simulink model "Final_Model_Building_2_AirflowAdded"  (R2022a)
settings: Solver=ode1  StartTime=0.0  StopTime=24*3600  FixedStep=10  RelTol=1e-3
values from neighbouring files (symbols this model uses):
  Aux_Threshold = 52    [Setup_Code_EWASP_VC.m]
  buildingAge = 2005    [Setup_Code_EWASP_VC.m]
  ceilingHeight = 2.4    [Setup_Code_EWASP_VC.m]
  conductiveHconnectMatrix = [ ... (first row only)    [Setup_Code_EWASP_VC.m]
  cRoofGreen = 100000    [Setup_Code_EWASP_VC.m]
  Defrost_After_Time = 30    [Setup_Code_EWASP_VC.m]
  DHWDemandProfile = occFreegainHotwaterElecTestPassiveOcc3(:,3)    [Setup_Code_EWASP_VC.m]
  Elec_Max = Elec_Max*(30/24.2)    [Setup_Code_EWASP_VC.m]
  Elec_Mid = Elec_Mid*(30/24.2)    [Setup_Code_EWASP_VC.m]
  Elec_Min = Elec_Min*(30/24.2)    [Setup_Code_EWASP_VC.m]
  ElecDemandProfile = occFreegainHotwaterElecTestPassiveOcc3(:,4)    [Setup_Code_EWASP_VC.m]
  ElecFixed = [Elec_Max(6,2) Elec_Max(6,4) Elec_Max(6,6) Elec_Max(6,7) ... (first row only)    [Setup_Code_EWASP_VC.m]
  floorOrCeilingArea = floorOrCeilingArea*1.15    [Setup_Code_EWASP_VC.m]
  forceCold = 0    [Setup_Code_EWASP_VC.m]
  freegain = occFreegainHotwaterElecTestPassiveOcc3(:,2)-max(occupancy)*25    [Setup_Code_EWASP_VC.m]
  furnitureModelOn = 1    [Setup_Code_EWASP_VC.m]
  Heat_Max = Heat_Max*(30/24.2)    [Setup_Code_EWASP_VC.m]
  Heat_Mid = Heat_Mid*(30/24.2)    [Setup_Code_EWASP_VC.m]
  Heat_Min = Heat_Min*(30/24.2)    [Setup_Code_EWASP_VC.m]
  HeatFixed = [Heat_Max(6,2) Heat_Max(6,4) Heat_Max(6,6) Heat_Max(6,7) ... (first row only)    [Setup_Code_EWASP_VC.m]
  HeatingOnProfile = repmat(HeatingOnProfile,365,1)    [Setup_Code_EWASP_VC.m]
  HEX_ReturnLowerLimit = 52.5    [Setup_Code_EWASP_VC.m]
  HEX_ReturnUpperLimit = 55    [Setup_Code_EWASP_VC.m]
  LeakMultiplier = 1+(2*(rand()-0.5)/10)    [Setup_Code_EWASP_VC.m]
  maxOcc = max(occupancyProfile)    [Setup_Code_EWASP_VC.m]
  NESW_wallArea = max(NESW_Lengths*ceilingHeight-NESW_Windows,0)    [Setup_Code_EWASP_VC.m]
  NESW_Windows = [ ... (first row only)    [Setup_Code_EWASP_VC.m]
  numRooms = roomCount    [Setup_Code_EWASP_VC.m]
  occupancy = occupancyProfile    [Setup_Code_EWASP_VC.m]
  offsetDays = 0    [Setup_Code_EWASP_VC.m]
  pumpChoice = pumpChoices(MinIndex,1)    [Setup_Code_EWASP_VC.m]
  pumpRamp = 180    [Setup_Code_EWASP_VC.m]
  ReturnLowerLimit = 37.5    [Setup_Code_EWASP_VC.m]
  ReturnUpperLimit = 40    [Setup_Code_EWASP_VC.m]
  RoofIrradiance = Flat_NS_EW_RoofIrradiance(:,1)    [Setup_Code_EWASP_VC.m]
  roofStartTemp = ones(11,1)*20    [Setup_Code_EWASP_VC.m]
  rooftype = 0    [Setup_Code_EWASP_VC.m]
  RoomDataMatrix = [zeros(1,12);ones(1,12)*wallDensity;zeros(1,12);ones(1,12)*wallU;ones(1,12)*windowU;ones(1,12)*floorU;ones(1,12)*ceilingU;zeros(1,12);windowArea, 0;floorOrCeilingArea;zeros(1,12);floorOrCeilingArea*ceilingHeight]    [Setup_Code_EWASP_VC.m]
  roomVol = roomVol*1.15    [Setup_Code_EWASP_VC.m]
  slabStartTemp = (GroundTempTimeSeries(offsetDays*1440+1,1)+thermostatSetting)/2    [Setup_Code_EWASP_VC.m]
  SlackRequest = zeros(1440,1)    [Setup_Code_EWASP_VC.m]
  SolarThermalExists = 0    [Setup_Code_EWASP_VC.m]
  SourceFixed = HeatFixed-ElecFixed    [Setup_Code_EWASP_VC.m]
  StateSeries = StateSeriesGenerator(22,7,1)    [Setup_Code_EWASP_VC.m]
  Tank_Lower_Temp = 49.5    [Setup_Code_EWASP_VC.m]
  Tank_Upper_Temp = 52    [Setup_Code_EWASP_VC.m]
  Tank_Volume_m3 = 0.15    [Setup_Code_EWASP_VC.m]
  TankHeatHour = randi([1 5])-1    [Setup_Code_EWASP_VC.m]
  upDown = [0;0;0;0;1;1;1;1;1;1;1]    [Setup_Code_EWASP_VC.m]
  wallStartTempExt = thermostatSetting*(0.266+0.00215*outdoorStartTemp+0.018*wallU+0.00113*outdoorStartTemp*wallU+0.0068*wallU^2)    [Setup_Code_EWASP_VC.m]
undefined symbols (not defined in the file or in its folder): a, ceilingU, condUDMatrix, convUDMatrix, deltaPEXPANDED_E, deltaPEXPANDED_E2, deltaPEXPANDED_N, deltaPEXPANDED_N2, deltaPEXPANDED_S, deltaPEXPANDED_S2, deltaPEXPANDED_W, deltaPEXPANDED_W2, DesiredDHWTemp, DesiredFlowTempVsInOutDeltaTemp, DiffuseHorizontal, DiscIntNeverNeededParam, DNI, dwnAndConcrete, DWORK_A_HX, DWORK_CHK_FLU, DWORK_CP_NODE, DWORK_DH, DWORK_FLUID, DWORK_HCON, DWORK_LOSS, DWORK_MDOTDOWN, DWORK_MDOTIN, DWORK_MDOTUP, DWORK_MIX, DWORK_PRESS, DWORK_QDOTIN, DWORK_RHO_NODE, DWORK_TIN, DWORK_TS_OLD, DWORK_V_NODE, ExtractRates, GroundTempTimeSeries, HCM, HCM2, HCM_closed, HCM_closed2, intermediateU, IsTop, massFlowMatrix, mechEfficiency, neighbourMatrix, numericalRoomUse, RadiatorMatrix, room2roomflowmatrix_E, room2roomflowmatrix_E2, room2roomflowmatrix_N, room2roomflowmatrix_N2, room2roomflowmatrix_S, room2roomflowmatrix_S2, room2roomflowmatrix_W, room2roomflowmatrix_W2, StateAirInEXPANDED_E, StateAirInEXPANDED_E2, StateAirInEXPANDED_N, StateAirInEXPANDED_N2 ... (+27)
libraries: simulink x6, dspsigops x4, dspmtrx3 x4, carnot x3, spsEdgeDetectorLib x2, dspstat3 x2, powerlib_meascontrol x1, simulink_extras x1
(part 2 of 27)

== system Final_Model_Building_2_AirflowAdded/Airflow Model ==
  note: Select the correct state solution from
      | the 2 states that are simulated
  In1 : Inport
  In2 : Inport  Port=2
  In3 : Inport  Port=3
  In4 : Inport  Port=4
  In5 : Inport  Port=5
  " output 1 - air is coming in output 2 - air is going out" : Subsystem
  Constant : Constant  Value=ExtractRates
  Constant1 : Constant  Value=occupancy
  Constant10 : Constant  Value=StateAirInEXPANDED_S
  Constant11 : Constant  Value=StateAirInEXPANDED_W
  Constant12 : Constant  Value=StateAirOutEXPANDED_S
  Constant13 : Constant  Value=StateAirOutEXPANDED_W
  Constant14 : Constant  Value=StateAirOutEXPANDED_N
  Constant15 : Constant  Value=StateAirOutEXPANDED_E
  Constant16 : Constant  Value=deltaPEXPANDED_N
  Constant17 : Constant  Value=deltaPEXPANDED_E
  Constant18 : Constant  Value=deltaPEXPANDED_S
  Constant19 : Constant  Value=deltaPEXPANDED_W
  Constant2 : Constant  Value=roomVol
  Constant20 : Constant  Value=numRooms
  Constant21 : Constant  Value=buildingAge
  Constant22 : Constant  Value=0
  Constant23 : Constant  Value=StateAirInEXPANDED_S2
  Constant24 : Constant  Value=StateAirInEXPANDED_W2
  Constant25 : Constant  Value=StateAirOutEXPANDED_S2
  Constant26 : Constant  Value=StateAirOutEXPANDED_W2
  Constant27 : Constant  Value=StateAirOutEXPANDED_N2
  Constant28 : Constant  Value=StateAirOutEXPANDED_E2
  Constant29 : Constant  Value=deltaPEXPANDED_N2
  Constant3 : Constant  Value=buildingAge
  Constant30 : Constant  Value=deltaPEXPANDED_E2
  Constant31 : Constant  Value=deltaPEXPANDED_S2
  Constant32 : Constant  Value=deltaPEXPANDED_W2
  Constant33 : Constant  Value=[0;0;0;0;0;0;0;0;0;0;0]
  Constant34 : Constant  Value=numRooms
  Constant35 : Constant  Value=[0;0;0;0;0;0;0;0;0;0;0]
  Constant36 : Constant  Value=room2roomflowmatrix_N2
  Constant37 : Constant  Value=room2roomflowmatrix_E2
  Constant38 : Constant  Value=room2roomflowmatrix_S2
  Constant39 : Constant  Value=room2roomflowmatrix_W2
  Constant4 : Constant  Value=room2roomflowmatrix_N
  Constant40 : Constant  Value=StateAirInEXPANDED_N2
  Constant41 : Constant  Value=StateAirInEXPANDED_E2
  Constant42 : Constant  Value=[0;0;0;0;0;0;0;0;0;0;0]
  Constant5 : Constant  Value=room2roomflowmatrix_E
  Constant6 : Constant  Value=room2roomflowmatrix_S
  Constant7 : Constant  Value=room2roomflowmatrix_W
  Constant8 : Constant  Value=StateAirInEXPANDED_N
  Constant9 : Constant  Value=StateAirInEXPANDED_E
  Corrected buoyancy2 : Display  Commented=on
  Corrected buoyancy3 : Display  Commented=on
  IsNaN : RelationalOperator  Operator=isNaN  OutDataTypeStr=boolean  RndMeth=Simplest  InputSameDT=off
  MATLAB Function : MATLAB Function  TreatAsAtomicUnit=on
  MATLAB Function1 : MATLAB Function  TreatAsAtomicUnit=on
  MATLAB Function2 : MATLAB Function  TreatAsAtomicUnit=on
  Mean : dspstat3/Mean  run=off  InputProcessing=Columns as channels (frame based)  reset_popup=None  directionMode=Each column  dimension=1  roiEnable=off  roiType=Rectangles  roiPortion=Entire ROI  roiOutput=Individual statistics for each ROI  roiFlag=off  roundingMode=Floor  overflowMode=off  outputDataTypeStr=Inherit: Same as accumulator  outputMin=[]  outputMax=[]  outputLastDataTypeStr=Inherit: Same as accumulator
  Offset Independent time series element selector2 : Subsystem
  Permute Dimensions : PermuteDimensions
  Plus{,2..3,5} (4 alike) : Sum
  Plus1 : Sum  Inputs=+-
  Plus4 : Sum  Inputs=+-
  Product1 : Product
  Product10 : Product  Inputs=*/
  Product2 : Product  Inputs=4
  Product3 : Product  Inputs=4
  Product4 : Product  Inputs=*/
  Product5 : Product  Inputs=**
  Product6 : Product  Inputs=**
  Product9 : Product
  Rate Transition{,1..5} (6 alike) : RateTransition  OutPortSampleTime=900
  Relay1 : Relay  OnSwitchValue=ThermostatSetting+1  OffSwitchValue=ThermostatSetting  OnOutputValue=0  OffOutputValue=1  OutDataTypeStr=boolean
  Selector{1..2,4..5,7,13..16} (9 alike) : Selector  NumberOfDimensions=2  InputPortWidth=3  IndexOptions=Index vector (dialog),Index vector (dialog)  Indices=1:numRooms,1  OutputSizes=1,1
  Selector10 : Selector  NumberOfDimensions=2  InputPortWidth=3  IndexOptions=Index vector (dialog),Index vector (dialog)  Indices=1:11,1  OutputSizes=1,1
  Selector{3,6,11..12} (4 alike) : Selector  NumberOfDimensions=2  InputPortWidth=3  IndexOptions=Index vector (dialog),Index vector (dialog)  Indices=1:numRooms,1:numRooms  OutputSizes=1,1
  Selector8 : Selector  NumberOfDimensions=2  InputPortWidth=3  IndexOptions=Index vector (dialog),Index vector (dialog)  Indices=1:11,1  OutputSizes=1,1
  Selector9 : Selector  NumberOfDimensions=2  InputPortWidth=3  IndexOptions=Index vector (dialog),Index vector (dialog)  Indices=1:11,1  OutputSizes=1,1
  StateLoader : MATLAB Function  TreatAsAtomicUnit=on
  StateLoader1 : MATLAB Function  TreatAsAtomicUnit=on
  Subsystem1 : Subsystem  TreatAsAtomicUnit=on  SystemSampleTime=10
      mask Display:
      | port_label('input', 1, 'R2R_flow_matrix')
      | port_label('input', 2, 'Between_Floor_dP')
      | port_label('input', 3, 'Air_out_vector')
      | port_label('input', 4, 'Air_In_Vector')
      | port_label('input', 5, 'Room_Temp_Vector')
      | port_label('input', 6, 'Outdoor_Air_Temp')
      | 
      | port_label('output', 1, 'room_Convective_Heat_Gain')
  Subsystem2 : Subsystem  TreatAsAtomicUnit=on  SystemSampleTime=10
      mask Display:
      | port_label('input', 1, 'R2R_flow_matrix')
      | port_label('input', 2, 'Between_Floor_dP')
      | port_label('input', 3, 'Air_out_vector')
      | port_label('input', 4, 'Air_In_Vector')
      | port_label('input', 5, 'Room_Temp_Vector')
      | port_label('input', 6, 'Outdoor_Air_Temp')
      | 
      | port_label('output', 1, 'room_Convective_Heat_Gain')
  Sum of Elements1 : Sum  Inputs=+
  Sum of Elements10 : Sum  Inputs=-
  Sum of Elements2 : Sum  Inputs=+  CollapseMode=Specified dimension
  Sum of Elements9 : Sum  Inputs=+
  Switch : Switch  Threshold=2020  SaturateOnIntegerOverflow=off  InputSameDT=off
  Switch1 : Switch  Threshold=2020  SaturateOnIntegerOverflow=off  InputSameDT=off
  Switch2 : Switch  Criteria=u2 > Threshold  Threshold=1.5  SaturateOnIntegerOverflow=off  InputSameDT=off
  Switch3 : Switch  Criteria=u2 > Threshold  Threshold=0.5  SaturateOnIntegerOverflow=off  InputSameDT=off
  Switch4 : Switch  Criteria=u2 > Threshold  Threshold=0.5  SaturateOnIntegerOverflow=off  InputSameDT=off
  Vector Concatenate : Concatenate
  Vector Concatenate1 : Concatenate
  Vector Concatenate2 : Concatenate
  heat capacity : Constant  Value=1000
  heat capacity1 : Constant  Value=1000
  oC to K : Constant  Value=273.15
  oC to K1 : Constant  Value=273.15
  oC to K2 : Constant  Value=mechEfficiency
  oC to K3 : Constant  Value=0
  Out1 : Outport  VectorParamsAs1DForOutWhenUnconnected=off
  TempFixForMechSystems : Outport  Port=2  VectorParamsAs1DForOutWhenUnconnected=off
  MinimumAirlossPhysicallyPossible : Outport  Port=3  VectorParamsAs1DForOutWhenUnconnected=off
  wires:
  [Wind_Speed] -> MATLAB Function/1(WindSpeed)
  Constant27/1 -> StateLoader1/12(StateAirOutEXPANDED_N)
  Selector1/1 -> [SAI_O]
  Constant15/1 -> StateLoader/13(StateAirOutEXPANDED_E)
  Constant19/1 -> StateLoader/19(deltaPEXPANDED_W)
  Constant9/1 -> StateLoader/9(StateAirInEXPANDED_E)
  Constant17/1 -> StateLoader/17(deltaPEXPANDED_E)
  Selector5/1 -> [SAO_O2]
  Constant26/1 -> StateLoader1/15(StateAirOutEXPANDED_W)
  Selector7/1 -> Corrected buoyancy3/1, Mean/1, [TVT]
  Subsystem1/1(Out1) -> Switch2/3
  Constant14/1 -> StateLoader/12(StateAirOutEXPANDED_N)
  Constant10/1 -> StateLoader/10(StateAirInEXPANDED_S)
  Subsystem2/1(Out1) -> Switch2/1
  [WindDir] -> MATLAB Function1/4(WindDir)
  [T_out] -> MATLAB Function1/3(T_out)
  StateLoader1/1(R2R_out) -> Selector11/1
  [Tin_Avg] -> MATLAB Function1/2(Tin_Avg)
  [R2R_Out] -> Subsystem1/1(In1)
  [Wind_Speed] -> MATLAB Function1/1(WindSpeed)
  Selector4/1 -> [SAI_O2]
  MATLAB Function1/3(DirIndex) -> StateLoader1/3(windDir)
  Constant31/1 -> StateLoader1/18(deltaPEXPANDED_S)
  Constant24/1 -> StateLoader1/11(StateAirInEXPANDED_W)
  MATLAB Function/2(StackIndex) -> Switch/3
  In4/1 -> [WindDir]
  Constant20/1 -> StateLoader/20(numRooms)
  Constant34/1 -> StateLoader1/20(numRooms)
  Constant5/1 -> StateLoader/5(room2roomflowmatrix_E)
  StateLoader1/2(StateAirIn_out) -> Selector13/1
  Constant6/1 -> StateLoader/6(room2roomflowmatrix_S)
  Constant38/1 -> StateLoader1/6(room2roomflowmatrix_S)
  [dP2] -> Subsystem2/2(In2)
  Constant29/1 -> StateLoader1/16(deltaPEXPANDED_N)
  Constant40/1 -> StateLoader1/8(StateAirInEXPANDED_N)
  Mean/1 -> [Tin_Avg], Corrected buoyancy2/1
  [WindDir] -> MATLAB Function/4(WindDir)
  Constant28/1 -> StateLoader1/13(StateAirOutEXPANDED_E)
  Constant32/1 -> StateLoader1/19(deltaPEXPANDED_W)
  Constant13/1 -> StateLoader/15(StateAirOutEXPANDED_W)
  [SAO_O] -> Subsystem1/3(In3)
  Constant36/1 -> StateLoader1/4(room2roomflowmatrix_N)
  Constant41/1 -> StateLoader1/9(StateAirInEXPANDED_E)
  [R2R_Out2] -> Subsystem2/1(In1)
  [SAO_O2] -> Subsystem2/3(In3)
  Constant23/1 -> StateLoader1/10(StateAirInEXPANDED_S)
  Constant30/1 -> StateLoader1/17(deltaPEXPANDED_E)
  Constant25/1 -> StateLoader1/14(StateAirOutEXPANDED_S)
  [SAI_O2] -> Subsystem2/4(In4)
  StateLoader1/4(deltaP) -> [dP2]
  Constant39/1 -> StateLoader1/7(room2roomflowmatrix_W)
  Constant8/1 -> StateLoader/8(StateAirInEXPANDED_N)
  Constant37/1 -> StateLoader1/5(room2roomflowmatrix_E)
  Selector6/1 -> [R2R_Out2]
  Constant12/1 -> StateLoader/14(StateAirOutEXPANDED_S)
  [dP] -> Subsystem1/2(In2)
  [T_out] -> Subsystem2/6(In6)
  MATLAB Function/1(WindIndex) -> StateLoader/1(windIndex)
  Constant7/1 -> StateLoader/7(room2roomflowmatrix_W)
  Constant16/1 -> StateLoader/16(deltaPEXPANDED_N)
  Selector2/1 -> [SAO_O]
  Constant4/1 -> StateLoader/4(room2roomflowmatrix_N)
  Constant11/1 -> StateLoader/11(StateAirInEXPANDED_W)
  [SAI_O] -> Subsystem1/4(In4)
  Selector3/1 -> [R2R_Out]
  Constant18/1 -> StateLoader/18(deltaPEXPANDED_S)
  MATLAB Function/3(DirIndex) -> StateLoader/3(windDir)
  [T_out] -> Subsystem1/6(In6)
  [Tin_Avg] -> MATLAB Function/2(Tin_Avg)
  [T_out] -> MATLAB Function/3(T_out)
  [TVT] -> Subsystem2/5(In5)
  In1/1 -> [Case_Switch]
  In2/1 -> [Wind_Speed]
  Switch2/1 -> Vector Concatenate/1
  In3/1 -> [T_out]
  In5/1 -> Selector7/1
  Constant35/1 -> Vector Concatenate/2
  Vector Concatenate/1 -> Selector8/1
  Selector8/1 -> Plus1/1
  Rate Transition/1 -> Selector2/1
  Rate Transition1/1 -> Selector3/1
  Rate Transition2/1 -> Selector1/1
  Rate Transition3/1 -> Selector6/1
  Rate Transition4/1 -> Selector4/1
  Rate Transition5/1 -> Selector5/1
  Constant2/1 -> MATLAB Function2/2(roomVol)
  Constant/1 -> MATLAB Function2/3(ExtractRates)
  heat capacity/1 -> Product2/4
  " output 1 - air is coming in output 2 - air is going out"/1(Out1) -> Product1/2, Product3/1
  [InsertTemp] -> Plus/2
  oC to K/1 -> Plus/1
  Plus/1 -> Product2/3
  [TVTex] -> Plus2/2
  oC to K1/1 -> Plus2/1
  Plus2/1 -> Product3/3
  heat capacity1/1 -> Product3/4
  Product3/1 -> Plus3/1
  Plus3/1 -> Plus1/2, Sum of Elements10/1
  MATLAB Function2/2(mechIndex) -> [mechIndex]
  [mechIndex] -> Switch/1
  Switch/1 -> StateLoader/2(stackIndex)
  Constant3/1 -> Switch/2
  MATLAB Function1/2(StackIndex) -> Switch1/3
  Switch1/1 -> StateLoader1/2(stackIndex)
  Constant21/1 -> Switch1/2
  [mechIndex] -> Switch1/1
  MATLAB Function1/1(WindIndex) -> StateLoader1/1(windIndex)
  [Case_Switch] -> Switch2/2
  Product1/1 -> Sum of Elements1/1, Product4/1
  Sum of Elements1/1 -> Product4/2
  Product4/1 -> Product5/1
  [TVTex] -> Product5/2
  Product5/1 -> Sum of Elements2/1
  Sum of Elements2/1 -> Switch3/3, IsNaN/1
  [ExtractTemp] -> Plus4/1
  [T_out] -> Plus4/2
  Plus4/1 -> Product6/1
  oC to K2/1 -> Switch4/1
  Product6/1 -> Plus5/1
  IsNaN/1 -> Switch3/2
  Constant22/1 -> Switch3/1
  Switch3/1 -> [ExtractTemp]
  [TVT] -> Vector Concatenate1/1
  Constant33/1 -> Vector Concatenate1/2
  Vector Concatenate1/1 -> Selector9/1
  Selector9/1 -> [TVTex]
  MATLAB Function2/1(y) -> Permute Dimensions/1
  Constant42/1 -> Vector Concatenate2/2
  Vector Concatenate2/1 -> Selector10/1
  Constant1/1 -> Offset Independent time series element selector2/1(In1)
  Offset Independent time series element selector2/1(Out1) -> MATLAB Function2/1(occupancy)
  oC to K3/1 -> Switch4/3
  Switch4/1 -> Product6/2
  [T_1] -> Relay1/1
  Relay1/1 -> Switch4/2
  Product2/1 -> Plus3/2
  Plus1/1 -> Out1/1
  Selector10/1 -> Product9/2, Product2/2, Product1/1, Product3/2, " output 1 - air is coming in output 2 - air is going out"/1(In1)
  " output 1 - air is coming in output 2 - air is going out"/2(Out2) -> Product9/1, Product2/1
  Plus5/1 -> [InsertTemp]
  [T_out] -> Plus5/2
  Product9/1 -> Sum of Elements9/1, Product10/1
  Sum of Elements9/1 -> Product10/2
  Product10/1 -> TempFixForMechSystems/1
  Sum of Elements10/1 -> MinimumAirlossPhysicallyPossible/1
  [TVT] -> Subsystem1/5(In5)
  Permute Dimensions/1 -> Vector Concatenate2/1
  Selector11/1 -> Rate Transition3/1
  StateLoader/1(R2R_out) -> Selector12/1
  StateLoader/4(deltaP) -> [dP]
  Selector12/1 -> Rate Transition1/1
  Selector13/1 -> Rate Transition4/1
  StateLoader1/3(StateAirOut_out) -> Selector14/1
  Selector14/1 -> Rate Transition5/1
  Selector15/1 -> Rate Transition/1
  StateLoader/3(StateAirOut_out) -> Selector15/1
  StateLoader/2(StateAirIn_out) -> Selector16/1
  Selector16/1 -> Rate Transition2/1

== system Final_Model_Building_2_AirflowAdded/CondLossIntermediate ==
  In1 : Inport
  Constant3 : Constant
  Constant5 : Constant  Value=intermediateU*ceilingHeight*conductiveHconnectMatrix'
  Constant6 : Constant
  Direct Lookup Table (n-D) : LookupNDDirect  InputsSelectThisObjectFromTable=Vector  TableIsInput=on
  Direct Lookup Table (n-D)1 : LookupNDDirect  NumberOfTableDimensions=1  TableIsInput=on
  Mux : Mux  Inputs=11
  Product2 : Product
  Subtract : Sum  Inputs=+-
  Subtract1 : Sum  Inputs=+-
  Subtract2 : Sum  Inputs=+-
  Sum of Elements : Sum  Inputs=+
  per room loss : Display
  temp diff : Display
  Out1 : Outport  VectorParamsAs1DForOutWhenUnconnected=off
  wires:
  [T_4] -> Mux/4
  [T_9] -> Mux/9
  In1/1 -> Subtract1/1, Subtract2/1
  Constant6/1 -> Subtract2/2
  Constant5/1 -> Direct Lookup Table (n-D)/2
  Product2/1 -> Sum of Elements/1, per room loss/1
  Direct Lookup Table (n-D)/1 -> Product2/1
  [T_2] -> Mux/2
  [T_6] -> Mux/6
  [T_7] -> Mux/7
  Direct Lookup Table (n-D)1/1 -> Subtract/2
  [T_5] -> Mux/5
  [T_10] -> Mux/10
  Constant3/1 -> Subtract1/2
  [T_8] -> Mux/8
  Subtract2/1 -> Direct Lookup Table (n-D)1/1
  Mux/1 -> Direct Lookup Table (n-D)1/2, Subtract/1
  [T_11] -> Mux/11
  Subtract/1 -> Product2/2, temp diff/1
  [T_3] -> Mux/3
  [T_1] -> Mux/1
  Subtract1/1 -> Direct Lookup Table (n-D)/1
  Sum of Elements/1 -> Out1/1

== system Final_Model_Building_2_AirflowAdded/GSHP_Subsystem ==
  note: Monitors for debugging
  Constant3 : Constant  Value=3600
  DHW for GSHP case : Subsystem
  Delay6 : Delay  DelayLength=5  InitialCondition=0
  Discrete-Time Integrator1 : DiscreteIntegrator  ExternalReset=falling  SampleTime=-1  LimitOutput=on  UpperSaturationLimit=1  LowerSaturationLimit=0  ICPrevOutput=DiscIntNeverNeededParam  ICPrevScaledInput=DiscIntNeverNeededParam
  Divide1 : Product  Inputs=*/
  Divide2 : Product  Inputs=*/
  Integrator14 : Integrator
  IsInf : RelationalOperator  Operator=isNaN  OutDataTypeStr=boolean  RndMeth=Simplest  InputSameDT=off
  Massflow when system is on12 : Constant  Value=3400/3600
  Plus : Sum
  Product : Product
  Product1 : Product
  Product3 : Product  Inputs=*/
  Scope21 : Scope
  Subsystem3 : Subsystem
      mask Display:
      | port_label('input', 1, 'T_Out')
      | port_label('input', 2, 'MixedTemp')
      | port_label('input', 3, 'MassFlowTotal')
      | port_label('input', 4, 'GCS')
      | port_label('input', 5, 'PowerFraction')
      | port_label('input', 6, 'DHW_on')
      | port_label('input', 7, 'ToGroundTot')
      | 
      | port_label('output', 1, 'Hysteresis')
      | port_label('output', 2, 'd_signal')
      | port_label('output', 3, 'THB_to_Pre')
      | 
      | port_label('output', 4, 'HeatToSpace')
      | port_label('output', 5, 'ElectrifiedHeatToSpace')
      | port_label('output', 6, 'ToGround')
      | port_label('output', 7, 'TotMdot')
      | 
      | disp('SH_GSHP')
  Sum : Sum  Inputs=|++
  Sum7 : Sum  Inputs=|++
  Switch2 : Switch  Criteria=u2 > Threshold  Threshold=0.5  SaturateOnIntegerOverflow=off  InputSameDT=off
  T_mains : Constant  Value=12
  Time in seconds for Heat pump to reach full stady state output1 : Constant  Value=180
  Water Demand Time Series (Minute)1 : Constant  Value=DHWDemandProfile
  tank_sensor_temp : Scope
  tag scope: AuxHeatToWater=global, DHW_on=global, ElectrifiedHeatToSpaceG=global, ElectrifiedHeatToWater=global, HeatToSpace=global, HeatToWater=global, THB_In_Pre=global, ToGround2=global, ToGround=global, ToGroundTot=global, TotMdot2=global, TotMdot=global, d_signal=global, d_signal_DHW=global, hysteresis=global, pump_power_Fraction=global
  wires:
  Product3/1 -> Switch2/3, IsInf/1
  Water Demand Time Series (Minute)1/1 -> DHW for GSHP case/5(In5)
  Subsystem3/4(Out4) -> [HeatToSpace]
  Integrator14/1 -> Scope21/1
  Divide2/1 -> Discrete-Time Integrator1/1
  DHW for GSHP case/1(Out1) -> tank_sensor_temp/1
  [d_signal] -> Plus/1
  DHW for GSHP case/2(Out2) -> [DHW_on]
  [MassFlowTotal] -> Subsystem3/3(In3)
  [DHW_on] -> Subsystem3/6(In6)
  [T_Out] -> Subsystem3/1(In1)
  DHW for GSHP case/7(Out7) -> [AuxHeatToWater]
  Discrete-Time Integrator1/1 -> Delay6/1
  [ToGround] -> Switch2/1, Product/1
  DHW for GSHP case/6(Out6) -> [HeatToWater]
  Subsystem3/3(Out3) -> [THB_In_Pre]
  [MixedTemp] -> Subsystem3/2(In2)
  Subsystem3/1(Out1) -> [hysteresis]
  [FromGround] -> DHW for GSHP case/1(In1)
  Plus/1 -> Divide2/1, Discrete-Time Integrator1/2
  Time in seconds for Heat pump to reach full stady state output1/1 -> Divide2/2
  [ToGround2] -> Product1/1
  [HeatToSpace] -> Divide1/1
  DHW for GSHP case/3(Out3) -> [ToGround2]
  [d_signal_DHW] -> Plus/2
  DHW for GSHP case/5(Out5) -> [ElectrifiedHeatToWater]
  Delay6/1 -> [pump_power_Fraction]
  Divide1/1 -> Integrator14/1
  [TotMdot] -> Product/2, Sum/1
  Product/1 -> Sum7/1
  DHW for GSHP case/4(Out4) -> [TotMdot2]
  Constant3/1 -> Divide1/2
  Subsystem3/7(Out7) -> [TotMdot]
  Massflow when system is on12/1 -> DHW for GSHP case/6(In6)
  DHW for GSHP case/8(Out8) -> [d_signal_DHW]
  [pump_power_Fraction] -> Subsystem3/5(In5)
  Subsystem3/6(Out6) -> [ToGround]
  Subsystem3/5(Out5) -> [ElectrifiedHeatToSpaceG]
  [ToGroundTot] -> Subsystem3/7(In7)
  Subsystem3/2(Out2) -> [d_signal]
  [Global_Control_Signal] -> Subsystem3/4(In4)
  [TotMdot2] -> Product1/2, Sum/2
  Sum/1 -> Product3/2
  [T_Out] -> DHW for GSHP case/3(In3)
  Product1/1 -> Sum7/2
  Sum7/1 -> Product3/1
  T_mains/1 -> DHW for GSHP case/4(In4)
  IsInf/1 -> Switch2/2
  Switch2/1 -> [ToGroundTot]
  [T_1] -> DHW for GSHP case/2(In2)
  Subsystem3/8(Out8) -> [FromGround]

== system Final_Model_Building_2_AirflowAdded/Offset Independent time series element selector ==
  In1 : Inport
  Clock1 : Clock
  Direct Lookup Table (n-D)1 : LookupNDDirect  NumberOfTableDimensions=1  TableIsInput=on
  Divide1 : Product  Inputs=*/
  Floor : Rounding
  Saturation2 : Saturate  UpperLimit=inf  LowerLimit=0
  Scope23 : Scope
  Sum : Sum  Inputs=|++
  on? (I/O)1 : Constant  Value=0  OutDataTypeStr=double
  on? (I/O)3 : Constant  Value=60  OutDataTypeStr=double
  Out1 : Outport  VectorParamsAs1DForOutWhenUnconnected=off
  wires:
  Saturation2/1 -> Scope23/1, Direct Lookup Table (n-D)1/1
  on? (I/O)3/1 -> Divide1/2
  Divide1/1 -> Floor/1
  Floor/1 -> Saturation2/1
  Clock1/1 -> Sum/1
  Direct Lookup Table (n-D)1/1 -> Out1/1
  In1/1 -> Direct Lookup Table (n-D)1/2
  on? (I/O)1/1 -> Sum/2
  Sum/1 -> Divide1/1

== system Final_Model_Building_2_AirflowAdded/Offset Independent time series element selector1 ==
  In1 : Inport
  Clock1 : Clock
  Direct Lookup Table (n-D)1 : LookupNDDirect  NumberOfTableDimensions=1  TableIsInput=on
  Divide1 : Product  Inputs=*/
  Floor : Rounding
  Saturation2 : Saturate  UpperLimit=inf  LowerLimit=0
  Scope23 : Scope
  Sum : Sum  Inputs=|++
  on? (I/O)2 : Constant  Value=offsetDays*3600*24  OutDataTypeStr=double
  on? (I/O)3 : Constant  Value=60  OutDataTypeStr=double
  Out1 : Outport  VectorParamsAs1DForOutWhenUnconnected=off
  wires:
  Saturation2/1 -> Scope23/1, Direct Lookup Table (n-D)1/1
  on? (I/O)3/1 -> Divide1/2
  Divide1/1 -> Floor/1
  Floor/1 -> Saturation2/1
  Clock1/1 -> Sum/1
  Direct Lookup Table (n-D)1/1 -> Out1/1
  In1/1 -> Direct Lookup Table (n-D)1/2
  Sum/1 -> Divide1/1
  on? (I/O)2/1 -> Sum/2

== system Final_Model_Building_2_AirflowAdded/Offset Independent time series element selector2 ==
  In1 : Inport
  Clock1 : Clock
  Direct Lookup Table (n-D)1 : LookupNDDirect  NumberOfTableDimensions=1  TableIsInput=on
  Divide1 : Product  Inputs=*/
  Floor : Rounding
  Saturation2 : Saturate  UpperLimit=inf  LowerLimit=0
  Scope23 : Scope
  Sum : Sum  Inputs=|++
  on? (I/O)1 : Constant  Value=0  OutDataTypeStr=double
  on? (I/O)3 : Constant  Value=60  OutDataTypeStr=double
  Out1 : Outport  VectorParamsAs1DForOutWhenUnconnected=off
  wires:
  Saturation2/1 -> Scope23/1, Direct Lookup Table (n-D)1/1
  on? (I/O)3/1 -> Divide1/2
  Divide1/1 -> Floor/1
  Floor/1 -> Saturation2/1
  Clock1/1 -> Sum/1
  Direct Lookup Table (n-D)1/1 -> Out1/1
  In1/1 -> Direct Lookup Table (n-D)1/2
  on? (I/O)1/1 -> Sum/2
  Sum/1 -> Divide1/1

== system Final_Model_Building_2_AirflowAdded/Radiator w//Thermostatic Control ==
  In1 : Inport
  In2 : Inport  Port=2
  In3 : Inport  Port=3
  1/(m*cp) : Gain  Gain=1/(Water_Volume*4180)  SaturateOnIntegerOverflow=on  OutDataTypeStr=Inherit: Same as input  ParamDataTypeStr=Inherit: Same as input
  Abs : Abs
  Add : Sum  Inputs=+-
  Constant : Constant  Value=4181
  Constant1 : Constant  Value=TRV_Therm_Setpoint
  Constant2 : Constant  Value=0.5
  Discrete-Time Integrator : DiscreteIntegrator  SampleTime=-1  ICPrevOutput=DiscIntNeverNeededParam  ICPrevScaledInput=DiscIntNeverNeededParam
  Divide : Product  Inputs=*/
  Divide1 : Product  Inputs=**
  Math Function : Math  Operator=pow  SignedPower=on
  Product : Product  Inputs=3  InputSameDT=on  SaturateOnIntegerOverflow=on  OutDataTypeStr=Inherit: Same as first input
  Product1 : Product  InputSameDT=on  SaturateOnIntegerOverflow=on  OutDataTypeStr=Inherit: Same as first input
  Product2 : Product
  Qdot2room1 : Scope
  Saturation : Saturate  UpperLimit=1  LowerLimit=0
  Scope : Scope
  Sign : Signum
  Sum : Sum  Inputs=-+  InputSameDT=on  SaturateOnIntegerOverflow=on  OutDataTypeStr=Inherit: Same as first input
  Sum1 : Sum  Inputs=-+  InputSameDT=on  SaturateOnIntegerOverflow=on  OutDataTypeStr=Inherit: Same as first input
  Sum2 : Sum
  Sum3 : Sum  Inputs=-+  InputSameDT=on  SaturateOnIntegerOverflow=on  OutDataTypeStr=Inherit: Same as first input
  Transfer Fcn (with initial states) : simulink_extras/Additional Linear/Transfer Fcn (with initial states)  Commented=on  N=[1]  D="[1  0]"  X0=20
  const : Constant  Value=1.3
  const1 : Constant  Value=Power_Nominal
  dTnom : Constant  Value=DeltaT_Nominal
  Out1 : Outport  VectorParamsAs1DForOutWhenUnconnected=off
  Out2 : Outport  Port=2  VectorParamsAs1DForOutWhenUnconnected=off
  Out3 : Outport  Port=3  VectorParamsAs1DForOutWhenUnconnected=off
  wires:
  Sum/1 -> Product/1
  Sum1/1 -> 1/(m*cp)/1
  Constant/1 -> Product/3
  Sum3/1 -> Sign/1, Divide/1
  const/1 -> Math Function/2
  Sign/1 -> Product1/2
  Product1/1 -> Out1/1, Sum1/1
  dTnom/1 -> Divide/2
  Abs/1 -> Math Function/1
  Product/1 -> Sum1/2
  In2/1 -> Sum/2
  const1/1 -> Divide1/2
  Divide1/1 -> Product1/1
  1/(m*cp)/1 -> Discrete-Time Integrator/1
  Math Function/1 -> Divide1/1
  Discrete-Time Integrator/1 -> Sum3/2, Sum/1, Scope/1, Out2/1
  Divide/1 -> Abs/1
  In1/1 -> Add/2, Sum3/1
  Product2/1 -> Product/2, Out3/1
  In3/1 -> Product2/1
  Constant1/1 -> Add/1
  Add/1 -> Sum2/1
  Constant2/1 -> Sum2/2
  Sum2/1 -> Saturation/1
  Saturation/1 -> Qdot2room1/1, Product2/2

== system Final_Model_Building_2_AirflowAdded/Select Correct Element from Array1 ==
  In1 : Inport
  Constant : Constant  Value=60
  Digital Clock : DigitalClock  SampleTime=10
  Direct Lookup Table (n-D) : LookupNDDirect  NumberOfTableDimensions=1  TableIsInput=on
  Divide : Product  Inputs=*/
  Floor : Rounding
  Saturation : Saturate  UpperLimit=inf  LowerLimit=0
  Out1 : Outport  VectorParamsAs1DForOutWhenUnconnected=off
  wires:
  Divide/1 -> Floor/1
  Saturation/1 -> Direct Lookup Table (n-D)/1
  Constant/1 -> Divide/2
  Floor/1 -> Saturation/1
  In1/1 -> Direct Lookup Table (n-D)/2
  Digital Clock/1 -> Divide/1
  Direct Lookup Table (n-D)/1 -> Out1/1

== system Final_Model_Building_2_AirflowAdded/Select Correct Element from Array2 ==
  In1 : Inport
  Constant : Constant  Value=60
  Digital Clock : DigitalClock  SampleTime=10
  Direct Lookup Table (n-D) : LookupNDDirect  NumberOfTableDimensions=1  TableIsInput=on
  Divide : Product  Inputs=*/
  Floor : Rounding
  Saturation : Saturate  UpperLimit=1439  LowerLimit=0
  Out1 : Outport  VectorParamsAs1DForOutWhenUnconnected=off
  wires:
  Divide/1 -> Floor/1
  Saturation/1 -> Direct Lookup Table (n-D)/1
  Constant/1 -> Divide/2
  Floor/1 -> Saturation/1
  In1/1 -> Direct Lookup Table (n-D)/2
  Digital Clock/1 -> Divide/1
  Direct Lookup Table (n-D)/1 -> Out1/1

== system Final_Model_Building_2_AirflowAdded/Select correct element from array, considering offset ==
  In1 : Inport
  Clock1 : Clock
  Direct Lookup Table (n-D)1 : LookupNDDirect  NumberOfTableDimensions=1  TableIsInput=on
  Divide1 : Product  Inputs=*/
  Floor : Rounding
  Saturation2 : Saturate  UpperLimit=inf  LowerLimit=0
  Scope23 : Scope
  Sum : Sum  Inputs=|++
  on? (I/O)1 : Constant  Value=offsetDays*3600*24  OutDataTypeStr=double
  on? (I/O)3 : Constant  Value=60  OutDataTypeStr=double
  Out1 : Outport  VectorParamsAs1DForOutWhenUnconnected=off
  wires:
  Saturation2/1 -> Scope23/1, Direct Lookup Table (n-D)1/1
  on? (I/O)3/1 -> Divide1/2
  Divide1/1 -> Floor/1
  Floor/1 -> Saturation2/1
  Clock1/1 -> Sum/1
  Direct Lookup Table (n-D)1/1 -> Out1/1
  In1/1 -> Direct Lookup Table (n-D)1/2
  on? (I/O)1/1 -> Sum/2
  Sum/1 -> Divide1/1

== system Final_Model_Building_2_AirflowAdded/Select correct element from array, considering offset1 ==
  In1 : Inport
  Clock1 : Clock
  Direct Lookup Table (n-D)1 : LookupNDDirect  NumberOfTableDimensions=1  TableIsInput=on
  Divide1 : Product  Inputs=*/
  Floor : Rounding
  Saturation2 : Saturate  UpperLimit=inf  LowerLimit=0
  Scope23 : Scope
  Sum : Sum  Inputs=|++
  on? (I/O)1 : Constant  Value=offsetDays*3600*24  OutDataTypeStr=double
  on? (I/O)3 : Constant  Value=60  OutDataTypeStr=double
  Out1 : Outport  VectorParamsAs1DForOutWhenUnconnected=off
  wires:
  Saturation2/1 -> Scope23/1, Direct Lookup Table (n-D)1/1
  on? (I/O)3/1 -> Divide1/2
  Divide1/1 -> Floor/1
  Floor/1 -> Saturation2/1
  Clock1/1 -> Sum/1
  Direct Lookup Table (n-D)1/1 -> Out1/1
  In1/1 -> Direct Lookup Table (n-D)1/2
  on? (I/O)1/1 -> Sum/2
  Sum/1 -> Divide1/1

== system Final_Model_Building_2_AirflowAdded/Select correct element from array, considering offset2 ==
  In1 : Inport
  Clock1 : Clock
  Direct Lookup Table (n-D)1 : LookupNDDirect  NumberOfTableDimensions=1  TableIsInput=on
  Divide1 : Product  Inputs=*/
  Floor : Rounding
  Saturation2 : Saturate  UpperLimit=inf  LowerLimit=0
  Scope23 : Scope
  Sum : Sum  Inputs=|++
  on? (I/O)1 : Constant  Value=offsetDays*3600*24  OutDataTypeStr=double
  on? (I/O)3 : Constant  Value=60  OutDataTypeStr=double
  Out1 : Outport  VectorParamsAs1DForOutWhenUnconnected=off
  wires:
  Saturation2/1 -> Scope23/1, Direct Lookup Table (n-D)1/1
  on? (I/O)3/1 -> Divide1/2
  Divide1/1 -> Floor/1
  Floor/1 -> Saturation2/1
  Clock1/1 -> Sum/1
  Direct Lookup Table (n-D)1/1 -> Out1/1
  In1/1 -> Direct Lookup Table (n-D)1/2
  on? (I/O)1/1 -> Sum/2
  Sum/1 -> Divide1/1

== system Final_Model_Building_2_AirflowAdded/Select correct element from array, considering offset3 ==
  In1 : Inport
  Clock1 : Clock
  Direct Lookup Table (n-D)1 : LookupNDDirect  NumberOfTableDimensions=1  TableIsInput=on
  Divide1 : Product  Inputs=*/
  Floor : Rounding
  Saturation2 : Saturate  UpperLimit=inf  LowerLimit=0
  Scope23 : Scope
  Sum : Sum  Inputs=|++
  on? (I/O)1 : Constant  Value=offsetDays*3600*24  OutDataTypeStr=double
  on? (I/O)3 : Constant  Value=60  OutDataTypeStr=double
  Out1 : Outport  VectorParamsAs1DForOutWhenUnconnected=off
  wires:
  Saturation2/1 -> Scope23/1, Direct Lookup Table (n-D)1/1
  on? (I/O)3/1 -> Divide1/2
  Divide1/1 -> Floor/1
  Floor/1 -> Saturation2/1
  Clock1/1 -> Sum/1
  Direct Lookup Table (n-D)1/1 -> Out1/1
  In1/1 -> Direct Lookup Table (n-D)1/2
  on? (I/O)1/1 -> Sum/2
  Sum/1 -> Divide1/1

== system Final_Model_Building_2_AirflowAdded/Select correct element from array, considering offset4 ==
  In1 : Inport
  Clock1 : Clock
  Direct Lookup Table (n-D)1 : LookupNDDirect  NumberOfTableDimensions=1  TableIsInput=on
  Divide1 : Product  Inputs=*/
  Floor : Rounding
  Saturation2 : Saturate  UpperLimit=inf  LowerLimit=0
  Scope23 : Scope
  Sum : Sum  Inputs=|++
  on? (I/O)1 : Constant  Value=offsetDays*3600*24  OutDataTypeStr=double
  on? (I/O)3 : Constant  Value=60  OutDataTypeStr=double
  Out1 : Outport  VectorParamsAs1DForOutWhenUnconnected=off
  wires:
  Saturation2/1 -> Scope23/1, Direct Lookup Table (n-D)1/1
  on? (I/O)3/1 -> Divide1/2
  Divide1/1 -> Floor/1
  Floor/1 -> Saturation2/1
  Clock1/1 -> Sum/1
  Direct Lookup Table (n-D)1/1 -> Out1/1
  In1/1 -> Direct Lookup Table (n-D)1/2
  on? (I/O)1/1 -> Sum/2
  Sum/1 -> Divide1/1

== system Final_Model_Building_2_AirflowAdded/Subsystem ==
  note: Bodged here - need to get a code that finds last non nan value
  In1 : Inport
  In2 : Inport  Port=2
  In3 : Inport  Port=3
  In4 : Inport  Port=4
  In5 : Inport  Port=5
  In6 : Inport  Port=6
  In7 : Inport  Port=7
  In8 : Inport  Port=8
  In9 : Inport  Port=9
  In10 : Inport  Port=10
  In11 : Inport  Port=11
  In12 : Inport  Port=12
  In13 : Inport  Port=13
  In14 : Inport  Port=14
  In15 : Inport  Port=15
  In16 : Inport  Port=16
  In17 : Inport  Port=17
  In18 : Inport  Port=18
  In19 : Inport  Port=19
  In20 : Inport  Port=20
  In21 : Inport  Port=21
  In22 : Inport  Port=22
  In23 : Inport  Port=23
  In24 : Inport  Port=24
  Add{1..4} (4 alike) : Sum  Inputs=12
  Ceil{,1..11} (12 alike) : Rounding  Operator=ceil
  Connect Count1 : Display
  Constant : Constant  Value=11
  Divide : Product  Inputs=*/
  IsNaN : RelationalOperator  Operator=isNaN  OutDataTypeStr=boolean  RndMeth=Simplest  InputSameDT=off
  "MassFlow. " : Display
  Product{,1..11} (12 alike) : Product
  Scope : Scope
  Scope1 : Scope
  Switch5 : Switch  Criteria=u2 > Threshold  Threshold=0.5  SaturateOnIntegerOverflow=off  InputSameDT=off
  positive delta T2 : Product  Inputs=*/
  Out1 : Outport  VectorParamsAs1DForOutWhenUnconnected=off
  Out2 : Outport  Port=2  VectorParamsAs1DForOutWhenUnconnected=off
  wires:
  Product5/1 -> Add2/6
  Product/1 -> Add2/1
  [SumUp12] -> Product11/1
  [SumUp9] -> Product8/1
  [SumUp9] -> Add1/9
  [SumUp7] -> Product6/1
  Product9/1 -> Add2/10
  [SumUp5] -> Product4/1
  [SumUp3] -> Add1/3
  In14/1 -> Add3/2, Product1/2
  In20/1 -> Add3/8, Product7/2
  Product8/1 -> Add2/9
  positive delta T2/1 -> Scope1/1, Switch5/3, Connect Count1/1, IsNaN/1
  [SumUp5] -> Add1/5
  Product1/1 -> Add2/2
  Product10/1 -> Add2/11
  [SumUp3] -> Product2/1
  Product6/1 -> Add2/7
  In15/1 -> Product2/2, Add3/3
  [SumUp4] -> Add1/4
  In17/1 -> Product4/2, Add3/5
  [SumUp2] -> Product1/1
  Add1/1 -> positive delta T2/2, Out1/1, "MassFlow. "/1
  In10/1 -> [SumUp10]
  [SumUp] -> Product/1
  [SumUp6] -> Product5/1
  In2/1 -> [SumUp2]
  Product4/1 -> Add2/5
  [SumUp6] -> Add1/6
  In24/1 -> Product11/2, Add3/12
  [SumUp11] -> Product10/1
  Product7/1 -> Add2/8
  Product3/1 -> Add2/4
  In18/1 -> Product5/2, Add3/6
  [SumUp7] -> Add1/7
  Product11/1 -> Add2/12
  [SumUp4] -> Product3/1
  In7/1 -> [SumUp7]
  Product2/1 -> Add2/3
  In23/1 -> Add3/11, Product10/2
  [SumUp11] -> Add1/11
  In16/1 -> Add3/4, Product3/2
  [SumUp10] -> Product9/1
  [SumUp12] -> Add1/12
  [SumUp10] -> Add1/10
  [SumUp2] -> Add1/2
  [SumUp] -> Add1/1
  In9/1 -> [SumUp9]
  [SumUp8] -> Product7/1
  In22/1 -> Product9/2, Add3/10
  Add2/1 -> positive delta T2/1
  [SumUp8] -> Add1/8
  In12/1 -> [SumUp12]
  In11/1 -> [SumUp11]
  In6/1 -> [SumUp6]
  In8/1 -> [SumUp8]
  In21/1 -> Add3/9, Product8/2
  In13/1 -> Add3/1, Product/2
  In19/1 -> Product6/2, Add3/7
  In5/1 -> [SumUp5]
  In3/1 -> [SumUp3]
  In4/1 -> [SumUp4]
  In1/1 -> [SumUp]
  Divide/1 -> Switch5/1
  IsNaN/1 -> Switch5/2
  Switch5/1 -> Out2/1
  Add3/1 -> Divide/1
  Constant/1 -> Divide/2
  [SumUp] -> Ceil/1
  [SumUp2] -> Ceil1/1
  [SumUp3] -> Ceil2/1
  [SumUp4] -> Ceil3/1
  [SumUp5] -> Ceil4/1
  [SumUp6] -> Ceil5/1
  [SumUp7] -> Ceil6/1
  [SumUp8] -> Ceil7/1
  [SumUp9] -> Ceil8/1
  [SumUp10] -> Ceil9/1
  [SumUp11] -> Ceil10/1
  [SumUp12] -> Ceil11/1
  Ceil/1 -> Add4/1
  Ceil1/1 -> Add4/2
  Ceil2/1 -> Add4/3
  Ceil3/1 -> Add4/4
  Ceil4/1 -> Add4/5
  Ceil5/1 -> Add4/6
  Ceil6/1 -> Add4/7
  Ceil7/1 -> Add4/8
  Ceil8/1 -> Add4/9
  Ceil9/1 -> Add4/10
  Ceil10/1 -> Add4/11
  Ceil11/1 -> Add4/12
  Add4/1 -> Scope/1

== system Final_Model_Building_2_AirflowAdded/Subsystem1 ==
  In1 : Inport
  In2 : Inport  Port=2
  In3 : Inport  Port=3
  In4 : Inport  Port=4
  In5 : Inport  Port=5
  In6 : Inport  Port=6
  In7 : Inport  Port=7
  In8 : Inport  Port=8
  In9 : Inport  Port=9
  In10 : Inport  Port=10
  In11 : Inport  Port=11
  In12 : Inport  Port=12
  In13 : Inport  Port=13
  Massflow when system is off{3..14} (12 alike) : Constant  Value=0
  Switch{7..18} (12 alike) : Switch  Criteria=u2 > Threshold  Threshold=0.5  SaturateOnIntegerOverflow=off  InputSameDT=off
  Out1 : Outport  VectorParamsAs1DForOutWhenUnconnected=off
  Out2 : Outport  Port=2  VectorParamsAs1DForOutWhenUnconnected=off
  Out3 : Outport  Port=3  VectorParamsAs1DForOutWhenUnconnected=off
  Out4 : Outport  Port=4  VectorParamsAs1DForOutWhenUnconnected=off
  Out5 : Outport  Port=5  VectorParamsAs1DForOutWhenUnconnected=off
  Out6 : Outport  Port=6  VectorParamsAs1DForOutWhenUnconnected=off
  Out7 : Outport  Port=7  VectorParamsAs1DForOutWhenUnconnected=off
  Out8 : Outport  Port=8  VectorParamsAs1DForOutWhenUnconnected=off
  Out9 : Outport  Port=9  VectorParamsAs1DForOutWhenUnconnected=off
  Out10 : Outport  Port=10  VectorParamsAs1DForOutWhenUnconnected=off
  Out11 : Outport  Port=11  VectorParamsAs1DForOutWhenUnconnected=off
  Out12 : Outport  Port=12  VectorParamsAs1DForOutWhenUnconnected=off
  wires:
  Massflow when system is off10/1 -> Switch11/3
  Switch9/1 -> Out3/1
  Switch7/1 -> Out1/1
  In1/1 -> Switch7/2, Switch9/2, Switch10/2, Switch17/2, Switch15/2, Switch18/2, Switch16/2, Switch11/2, Switch14/2, Switch13/2, Switch12/2, Switch8/2
  Massflow when system is off5/1 -> Switch9/3
  In4/1 -> Switch9/1
  Massflow when system is off6/1 -> Switch10/3
  Switch11/1 -> Out8/1
  Switch14/1 -> Out7/1
  Massflow when system is off11/1 -> Switch16/3
  Massflow when system is off9/1 -> Switch14/3
  Massflow when system is off13/1 -> Switch18/3
  Switch15/1 -> Out12/1
  Switch10/1 -> Out4/1
  Switch17/1 -> Out10/1
  Massflow when system is off3/1 -> Switch7/3
  Massflow when system is off4/1 -> Switch8/3
  Massflow when system is off14/1 -> Switch15/3
  In12/1 -> Switch18/1
  Massflow when system is off12/1 -> Switch17/3
  In7/1 -> Switch13/1
  Switch12/1 -> Out5/1
  In5/1 -> Switch10/1
  Massflow when system is off8/1 -> Switch13/3
  Massflow when system is off7/1 -> Switch12/3
  In11/1 -> Switch17/1
  Switch18/1 -> Out11/1
  In9/1 -> Switch11/1
  Switch13/1 -> Out6/1
  In3/1 -> Switch8/1
  In2/1 -> Switch7/1
  Switch16/1 -> Out9/1
  In13/1 -> Switch15/1
  In10/1 -> Switch16/1
  In6/1 -> Switch12/1
  In8/1 -> Switch14/1
  Switch8/1 -> Out2/1

== system Final_Model_Building_2_AirflowAdded/Subsystem2 ==
  note: last off
  In1 : Inport
  Clock : Clock
  Clock1 : Clock
  Clock3 : Clock
  Delay1 : Delay  DelayLength=1  InitialCondition=0
  Delay2 : Delay  DelayLength=1  InitialCondition=0
  Ground : Ground
  Logical Operator1 : Logic  AllPortsSameDT=off  OutDataTypeStr=boolean
  Logical Operator2 : Logic  Operator=NOT  AllPortsSameDT=off  OutDataTypeStr=boolean
  Logical Operator3 : Logic  AllPortsSameDT=off  OutDataTypeStr=boolean
  Logical Operator4 : Logic  Operator=NOT  AllPortsSameDT=off  OutDataTypeStr=boolean
  Memory : Memory
  Sample and Hold : dspsigops/Sample and Hold  trig=Rising edge  initCond=0  latchinput=off
  Sample and Hold1 : dspsigops/Sample and Hold  trig=Rising edge  initCond=0  latchinput=off
  Scope20 : Scope  NumInputPorts=2
  Scope21 : Scope
  Subtract : Sum  Inputs=-+
  Subtract1 : Sum  Inputs=+-
  Switch2 : Switch  Criteria=u2 > Threshold  SaturateOnIntegerOverflow=off  InputSameDT=off
  Switch3 : Switch  Threshold=1  SaturateOnIntegerOverflow=off  InputSameDT=off
  Switch4 : Switch  Criteria=u2 > Threshold  Threshold=600  SaturateOnIntegerOverflow=off  InputSameDT=off
  on? (I/O)3 : Constant  OutDataTypeStr=double
  on? (I/O)4 : Constant  Value=0  OutDataTypeStr=double
  on? (I/O)5 : Constant  OutDataTypeStr=double
  on? (I/O)6 : Constant  OutDataTypeStr=double
  on? (I/O)7 : Constant  Value=0  OutDataTypeStr=double
  Out1 : Outport  VectorParamsAs1DForOutWhenUnconnected=off
  wires:
  Clock3/1 -> Sample and Hold/1
  Sample and Hold/1 -> Subtract/2
  Logical Operator1/1 -> Sample and Hold1/Trigger
  Delay1/1 -> Logical Operator2/1
  In1/1 -> Logical Operator1/1, Delay1/1, Delay2/1, Logical Operator4/1
  [on_time] -> Subtract1/2
  on? (I/O)3/1 -> Switch2/1
  Sample and Hold1/1 -> [on_time], Scope20/1, Subtract/1
  on? (I/O)7/1 -> Switch4/3
  Delay2/1 -> Logical Operator3/2
  Logical Operator2/1 -> Logical Operator1/2
  Switch4/1 -> Switch3/1
  Logical Operator3/1 -> Sample and Hold/Trigger
  Clock/1 -> Sample and Hold1/1
  Logical Operator4/1 -> Logical Operator3/1
  on? (I/O)6/1 -> Switch4/1
  Subtract1/1 -> Switch4/2
  Subtract/1 -> Switch2/2
  on? (I/O)5/1 -> Switch3/3
  Memory/1 -> Out1/1
  Switch3/1 -> Memory/1
  on? (I/O)4/1 -> Switch2/3
  Clock1/1 -> Subtract1/1
  Ground/1 -> Scope20/2
  Switch2/1 -> Scope21/1, Switch3/2

== system Final_Model_Building_2_AirflowAdded/Subsystem3 ==
  note: roof masses (45kg/m^2) and heat capacities calculated
      | using https://www.steelbeamcalculator.co.uk/standardloads
  In1 : Inport
  In2 : Inport  Port=2
  In3 : Inport  Port=3
  Ceil node tmperatures : DiscreteIntegrator  InitialConditionSource=external  InitialCondition=20  SampleTime=-1  ICPrevOutput=DiscIntNeverNeededParam  ICPrevScaledInput=DiscIntNeverNeededParam
  Display1 : Display
  Divide : Product  Inputs=*/
  Divide1 : Product  Inputs=*/
  Heat to ceilingNodes : Product  Inputs=4
  Heat to roofspace airnode : Sum  Inputs=+
  Heatloss roof to environment : Subsystem
  MATLAB Function1 : MATLAB Function  TreatAsAtomicUnit=on
  MATLAB Function2 : MATLAB Function  TreatAsAtomicUnit=on
  MATLAB Function3 : MATLAB Function  TreatAsAtomicUnit=on
  MATLAB Function4 : MATLAB Function  TreatAsAtomicUnit=on
  Product1 : Product  Inputs=3
  "Roof Temp " : DiscreteIntegrator  InitialConditionSource=external  InitialCondition=20  SampleTime=-1  ICPrevOutput=DiscIntNeverNeededParam  ICPrevScaledInput=DiscIntNeverNeededParam
  "RoofspaceTemp " : DiscreteIntegrator  InitialConditionSource=external  InitialCondition=20  SampleTime=-1  ICPrevOutput=DiscIntNeverNeededParam  ICPrevScaledInput=DiscIntNeverNeededParam
  Subtract : Sum  Inputs=+-
  Subtract1 : Sum
  Subtract2 : Sum  Inputs=+-
  Subtract3 : Sum  Inputs=+-
  Subtract4 : Sum  Inputs=2
  Subtract5 : Sum  Inputs=-+
  Total roofstructure heat capacity : Product
  Unary Minus : UnaryMinus
  air density per m3 : Constant  Value=1.225
  air heat capacity per kg : Constant  Value=1000
  ceiling heatchange due to loss to roofspace : UnaryMinus
  ceilnode heat capacities(predominantly plaster mass) : Constant  Value=10*1090*(IsTop(1:1:11)').*floorOrCeilingArea(1:1:11)'
  ceilnode heat capacities(predominantly plaster mass)1 : Constant  Value=10*1090*(IsTop(1,1:11)').*floorOrCeilingArea(1,1:11)'
  convective transfer to ceiling node : Constant  Value=2
  deltaTCeilingNodes : Product  Inputs=*/
  deltaTCeilingNodes1 : Product  Inputs=*/
  estimate of pitched roofspace air volume: 0.5 * floorArea of loft * height at peak : Constant  Value=0.5*sum(floorOrCeilingArea(1,1:11)'.*IsTop(1,1:11)')*(0.5*(sum(floorOrCeilingArea(1,1:11)'.*IsTop(1,1:11)')).^0.5)
  heat loss ceiing to roofspace : Product
  heat loss roofspace to roof : Product
  initial ceilnode temps : Constant  Value=20*ones(11,1)
  initial ceilnode temps1 : Constant  Value=10
  initial ceilnode temps2 : Constant  Value=10
  mass of roof per m^2*predictedroofarea : Constant  Value=45*sum(floorOrCeilingArea(1,1:11)'.*IsTop(1,1:11)')*1.414
  roofspace heatchange due to loss to roof : UnaryMinus
  room is on the top floor : Constant  Value=IsTop(1,1:11)'
  room is on the top floor1 : Constant  Value=floorOrCeilingArea(1,1:11)'
  slate heat capacity per kg1 : Constant  Value=760
  w/k loss from ceiling to roofspace : Constant  Value=(ceilingU*2)*(floorOrCeilingArea(1,1:11)').*(IsTop(1,1:11)')
  w/k loss from roofspace to roof : Constant  Value=(ceilingU*2)*sum(floorOrCeilingArea(1,1:11)'.*IsTop(1,1:11)')*1.414
  Out1 : Outport  VectorParamsAs1DForOutWhenUnconnected=off
  wires:
  In2/1 -> [windSpeed]
  In1/1 -> Subtract/1
  Subtract5/1 -> Divide1/1
  w/k loss from roofspace to roof/1 -> heat loss roofspace to roof/2
  Subtract/1 -> Heat to ceilingNodes/1
  Product1/1 -> Divide/2
  estimate of pitched roofspace air volume: 0.5 * floorArea of loft * height at peak/1 -> Product1/2
  air heat capacity per kg/1 -> Product1/3
  room is on the top floor/1 -> Heat to ceilingNodes/2
  heat loss roofspace to roof/1 -> roofspace heatchange due to loss to roof/1, Subtract5/2
  MATLAB Function3/1(y) -> Subtract1/2
  convective transfer to ceiling node/1 -> Heat to ceilingNodes/4
  air density per m3/1 -> Product1/1
  initial ceilnode temps1/1 -> "RoofspaceTemp "/2
  Heatloss roof to environment/1(Out1) -> Subtract5/1
  Heat to roofspace airnode/1 -> Display1/1, Subtract4/1
  Total roofstructure heat capacity/1 -> Divide1/2
  slate heat capacity per kg1/1 -> Total roofstructure heat capacity/1
  deltaTCeilingNodes1/1 -> MATLAB Function3/1(u)
  ceilnode heat capacities(predominantly plaster mass)1/1 -> deltaTCeilingNodes1/2
  MATLAB Function4/1(y) -> "Roof Temp "/1
  w/k loss from ceiling to roofspace/1 -> heat loss ceiing to roofspace/2
  deltaTCeilingNodes/1 -> MATLAB Function1/1(u)
  Subtract4/1 -> Divide/1
  Subtract3/1 -> heat loss roofspace to roof/1
  MATLAB Function2/1(y) -> "RoofspaceTemp "/1
  room is on the top floor1/1 -> Heat to ceilingNodes/3
  Ceil node tmperatures/1 -> Subtract2/1, Subtract/2
  mass of roof per m^2*predictedroofarea/1 -> Total roofstructure heat capacity/2
  ceilnode heat capacities(predominantly plaster mass)/1 -> deltaTCeilingNodes/2
  ceiling heatchange due to loss to roofspace/1 -> deltaTCeilingNodes1/1
  [windSpeed] -> Heatloss roof to environment/1(In1)
  initial ceilnode temps2/1 -> "Roof Temp "/2
  Heat to ceilingNodes/1 -> Unary Minus/1, deltaTCeilingNodes/1
  MATLAB Function1/1(y) -> Subtract1/1
  In3/1 -> [outdoorTemp]
  roofspace heatchange due to loss to roof/1 -> Subtract4/2
  Subtract2/1 -> heat loss ceiing to roofspace/1
  Divide1/1 -> MATLAB Function4/1(u)
  Divide/1 -> MATLAB Function2/1(u)
  "RoofspaceTemp "/1 -> Subtract3/1, Subtract2/2
  [outdoorTemp] -> Heatloss roof to environment/2(In2)
  Subtract1/1 -> Ceil node tmperatures/1
  initial ceilnode temps/1 -> Ceil node tmperatures/2
  heat loss ceiing to roofspace/1 -> ceiling heatchange due to loss to roofspace/1, Heat to roofspace airnode/1
  "Roof Temp "/1 -> Subtract3/2, Heatloss roof to environment/3(In3)
  Unary Minus/1 -> Out1/1

== system Final_Model_Building_2_AirflowAdded/Subsystem4 ==
  In1 : Inport
  Constant13 : Constant  Value=5
  "Select correct element from array, considering offset6" : Subsystem
  multiplication accounts for input data # being scaled 5 times too small : Product  Inputs=**
  Out1 : Outport  VectorParamsAs1DForOutWhenUnconnected=off
  wires:
  "Select correct element from array, considering offset6"/1(Out1) -> multiplication accounts for input data # being scaled 5 times too small/1
  In1/1 -> "Select correct element from array, considering offset6"/1(In1)
  Constant13/1 -> multiplication accounts for input data # being scaled 5 times too small/2
  multiplication accounts for input data # being scaled 5 times too small/1 -> Out1/1
